simulink model "BLDCmotorControl_FOC_R2017b_fixdt"  (R2017b)
settings: Solver=FixedStepDiscrete  StartTime=0  StopTime=0.5  FixedStep=Ts  MaxStep=1e-6  RelTol=1e-6  AbsTol=1e-6  EnableMultiTasking=on
PreLoadFcn:
  | addpath(pwd);
  | addpath(genpath('01_Libraries'));
  | addpath(genpath('02_Figures'));
  | addpath(genpath('03_CreateParamTable'));
InitFcn:
  | init_model;
values from neighbouring files (symbols this model uses):
  a_elecAngle = 60    [init_model.m]
  a_elecPeriod = 360    [init_model.m]
  a_phaAdvMax = 25    [init_model.m]
  b_diagEna = 1    [init_model.m]
  b_fieldWeakEna = 0    [init_model.m]
  cf_currFilt = 0.12    [init_model.m]
  cf_idKi = 60 / (f_ctrl/3)    (= 0.01125)    [init_model.m]
  cf_idKp = 0.2    [init_model.m]
  cf_iqKi = 100 / (f_ctrl/3)    (= 0.01875)    [init_model.m]
  cf_iqKiLimProt = 60 / (f_ctrl/3)    (= 0.01125)    [init_model.m]
  cf_iqKp = 0.3    [init_model.m]
  cf_KbLimProt = 1000 / (f_ctrl/3)    (= 0.1875)    [init_model.m]
  cf_nKi = 20.4 / (f_ctrl/3)    (= 0.003825)    [init_model.m]
  cf_nKiLimProt = 20 / (f_ctrl/3)    (= 0.00375)    [init_model.m]
  cf_nKp = 1.18    [init_model.m]
  cf_speedCoef = round(f_ctrl * a_mechAngle * (pi/180) * (30/pi))    [init_model.m]
  CTRL_COM = 0    [init_model.m]
  CTRL_FOC = 2    [init_model.m]
  CTRL_SIN = 1    [init_model.m]
  dV_openRate = 1000 / (f_ctrl/3)    (= 0.1875)    [init_model.m]
  dz_cntTrnsDetHi = 40    [init_model.m]
  dz_cntTrnsDetLo = 20    [init_model.m]
  i_max = i_max * i_sca    (= 750)    [init_model.m]
  id_fieldWeakMax = 5 * i_sca    (= 250)    [init_model.m]
  iq_maxSca_M1 = sqrt(1 - iq_maxSca_XA.^2)    [init_model.m]
  n_commAcvLo = 15    [init_model.m]
  n_commDeacvHi = 30    [init_model.m]
  n_fieldWeakAuthHi = 400    [init_model.m]
  n_fieldWeakAuthLo = 300    [init_model.m]
  n_max = 1000    [init_model.m]
  n_polePairs = 15    [init_model.m]
  n_stdStillDet = 3    [init_model.m]
  OPEN_MODE = 0    [init_model.m]
  r_cos_M1 = cos((a_elecAngle_XA + 0)*(pi/180))    [init_model.m]
  r_errInpTgtThres = 600    [init_model.m]
  r_fieldWeakHi = 1500    [init_model.m]
  r_fieldWeakLo = 1000    [init_model.m]
  r_sin3PhaA_M1 = sin3Arm + A*r_sinPhaA_M1    [init_model.m]
  r_sin3PhaB_M1 = sin3Arm + A*r_sinPhaB_M1    [init_model.m]
  r_sin3PhaC_M1 = sin3Arm + A*r_sinPhaC_M1    [init_model.m]
  r_sin_M1 = sin((a_elecAngle_XA + 0)*(pi/180))    [init_model.m]
  SPD_MODE = 2    [init_model.m]
  t_errDequal = 1.80 * f_ctrl/3    (= 9600)    [init_model.m]
  t_errQual = 0.24 * f_ctrl/3    (= 1280)    [init_model.m]
  TRQ_MODE = 3    [init_model.m]
  Ts = 5e-6    (= 5e-06)    [init_model.m]
  Ts_ctrl = 6e-5    (= 6e-05)    [init_model.m]
  Vd_max = 1000 - V_margin    (= 900)    [init_model.m]
  vec_hallToPos = [0 2 0 1 4 3 5 0]    [init_model.m]
  VLT_MODE = 1    [init_model.m]
  Vq_max_M1 = sqrt(Vd_max^2 - Vq_max_XA.^2)    [init_model.m]
  z_commutMap_M1 = [-1 -1  0  1  1  0 ... (first row only)    [init_model.m]
  z_ctrlModReq = VLT_MODE    (= 1)    [init_model.m]
  z_ctrlTypSel = 2    [init_model.m]
  z_maxCntRst = 2000    [init_model.m]
  z_selPhaCurMeasABC = 0    [init_model.m]
undefined symbols (not defined in the file or in its folder): DiscIntNeverNeededParam, sigbuilder_block
libraries: BLDC_controller_Lib x15, simulink x14, powerlib x6, pePwmGenerator x1
(part 2 of 4)

== system BLDCmotorControl_FOC_R2017b_fixdt/rateLimiter ==
  u : Inport
  rate : Inport  Port=2
  Data Type Conversion1 : DataTypeConversion  OutDataTypeStr=fixdt(1,16,4)
  Gain : Gain  Tag=struct('comment',struct('text','','placement',1),'logdata',struct('maxnumvals',inf,'plotchannels',[],'loggingmode',3,'channels',1),'output',struct('variable','','description','','name','$S_$B','width',1,'address','','max',NaN,'min',NaN,'class','default','type','CONTINUOUS','scaling','','lsb',1,'offset',0,'arb',0,'freeze',1,'unit','','autoscalingmode',1,'lowerheadroom',1,'upperheadroom',1,'headroomunit','bit','keepdatatype',1,'checkmin',0,'checkmax',0,'castoutput',0,'show',0),'gain',struct('variable','','description','','name','$S_$B_gain','width',1,'address','','max',NaN,'min',NaN,'class','default','type','CONTINUOUS','scaling','','lsb',1,'offset',0,'arb',0,'freeze',1,'unit','','keepdatatype',1,'value','1','scalar',0,'tolerance',1),'scalingvalid',0,'date',730486)  Gain=-1  RndMeth=Zero  OutDataTypeStr=Inherit: Same as input  ParamDataTypeStr=Inherit: Same as input
  Rate_Limiter : Subsystem
      settings: RTWFcnNameOpts=Use subsystem name
      mask Display: plot([0.15 0.85],[0.5 0.5],[0.5 0.5],[0.1 0.9],[0.25 0.75],[0.1 0.9])
  y : Outport
  wires:
  Data Type Conversion1/1 -> Rate_Limiter/1(u)
  u/1 -> Data Type Conversion1/1
  Rate_Limiter/1(y) -> y/1
  rate/1 -> Gain/1, Rate_Limiter/2(inc)
  Gain/1 -> Rate_Limiter/3(dec)

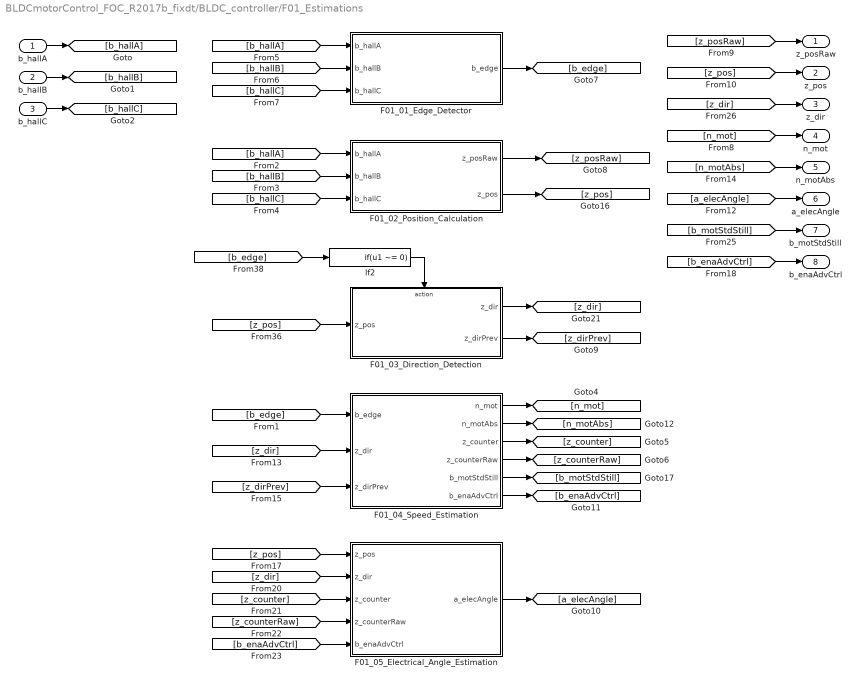
== system BLDCmotorControl_FOC_R2017b_fixdt/BLDC_controller/F01_Estimations ==
  b_hallA : Inport
  b_hallB : Inport  Port=2
  b_hallC : Inport  Port=3
  F01_01_Edge_Detector : Subsystem
  F01_02_Position_Calculation : Subsystem
  F01_03_Direction_Detection : Subsystem
  F01_04_Speed_Estimation : Subsystem
  F01_05_Electrical_Angle_Estimation : Subsystem
  If2 : If  IfExpression=u1 ~= 0  ShowElse=off
  z_posRaw : Outport  OutputWhenDisabled=reset  InitialOutput=0
  z_pos : Outport  Port=2  OutputWhenDisabled=reset  InitialOutput=0
  z_dir : Outport  Port=3  OutputWhenDisabled=reset  InitialOutput=0
  "n_mot " : Outport  Port=4  OutputWhenDisabled=reset  InitialOutput=0
  n_motAbs : Outport  Port=5  OutputWhenDisabled=reset  InitialOutput=0
  a_elecAngle : Outport  Port=6  OutputWhenDisabled=reset  InitialOutput=0
  b_motStdStill : Outport  Port=7  OutputWhenDisabled=reset  InitialOutput=0
  b_enaAdvCtrl : Outport  Port=8
  wires:
  If2/1 -> F01_03_Direction_Detection/Action
  [b_edge] -> If2/1
  [z_pos] -> F01_03_Direction_Detection/1(z_pos)
  [b_hallA] -> F01_01_Edge_Detector/1(b_hallA)
  F01_01_Edge_Detector/1("b_edge ") -> [b_edge]
  F01_03_Direction_Detection/1(z_dir) -> [z_dir]
  [b_hallB] -> F01_01_Edge_Detector/2(b_hallB)
  [b_hallC] -> F01_01_Edge_Detector/3(b_hallC)
  b_hallA/1 -> [b_hallA]
  b_hallB/1 -> [b_hallB]
  b_hallC/1 -> [b_hallC]
  [b_hallC] -> F01_02_Position_Calculation/3(b_hallC)
  [b_hallB] -> F01_02_Position_Calculation/2(b_hallB)
  [b_hallA] -> F01_02_Position_Calculation/1(b_hallA)
  F01_02_Position_Calculation/2("z_pos ") -> [z_pos]
  [b_edge] -> F01_04_Speed_Estimation/1(b_edge)
  F01_04_Speed_Estimation/1(n_mot) -> [n_mot]
  [n_mot] -> "n_mot "/1
  [z_pos] -> z_pos/1
  [z_dir] -> F01_04_Speed_Estimation/2(z_dir)
  F01_04_Speed_Estimation/3(z_counter) -> [z_counter]
  F01_04_Speed_Estimation/4(z_counterRaw) -> [z_counterRaw]
  F01_03_Direction_Detection/2(z_dirPrev) -> [z_dirPrev]
  [z_dirPrev] -> F01_04_Speed_Estimation/3(z_dirPrev)
  [z_pos] -> F01_05_Electrical_Angle_Estimation/1(z_pos)
  [z_dir] -> F01_05_Electrical_Angle_Estimation/2(z_dir)
  [z_counter] -> F01_05_Electrical_Angle_Estimation/3(z_counter)
  [z_counterRaw] -> F01_05_Electrical_Angle_Estimation/4(z_counterRaw)
  [b_enaAdvCtrl] -> F01_05_Electrical_Angle_Estimation/5(b_enaAdvCtrl)
  F01_04_Speed_Estimation/6(b_enaAdvCtrl) -> [b_enaAdvCtrl]
  [b_enaAdvCtrl] -> b_enaAdvCtrl/1
  [a_elecAngle] -> a_elecAngle/1
  F01_05_Electrical_Angle_Estimation/1(a_elecAngle) -> [a_elecAngle]
  F01_04_Speed_Estimation/2(n_motAbs) -> [n_motAbs]
  [n_motAbs] -> n_motAbs/1
  F01_02_Position_Calculation/1(z_posRaw) -> [z_posRaw]
  [z_posRaw] -> z_posRaw/1
  [b_motStdStill] -> b_motStdStill/1
  F01_04_Speed_Estimation/5(b_motStdStill) -> [b_motStdStill]
  [z_dir] -> z_dir/1

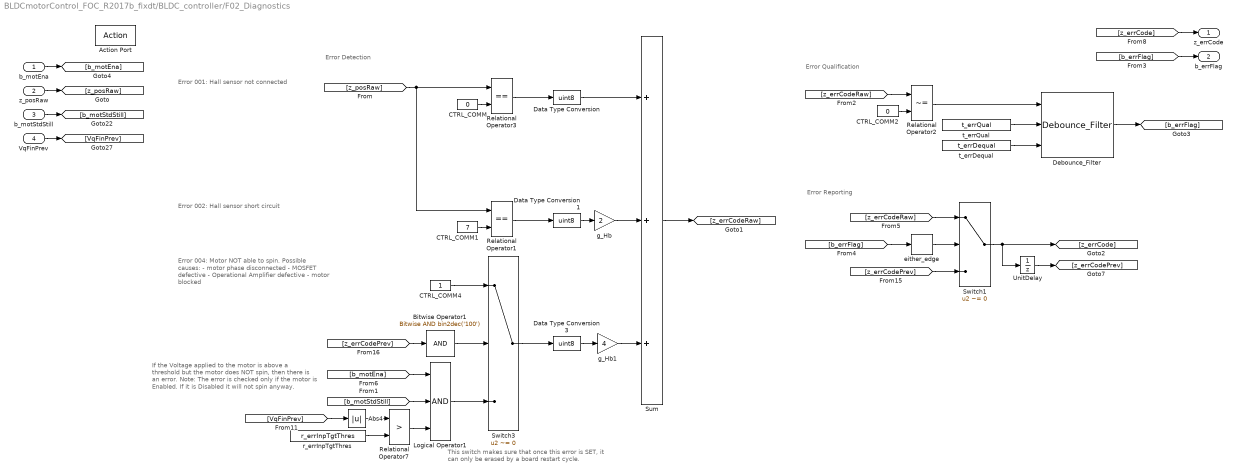
== system BLDCmotorControl_FOC_R2017b_fixdt/BLDC_controller/F02_Diagnostics ==
  note: Error 001: Hall sensor not connected
  note: Error 002: Hall sensor short circuit
  note: Error Qualification
  note: Error Detection
  note: Error Reporting
  note: Error 004: Motor NOT able to spin.
      |
      | Possible causes:
      | - motor phase disconnected
      | - MOSFET defective
      | - Operational Amplifier defective
      | - motor blocked
  note: This switch makes sure that once this error is SET, it can only be erased by a board restart cycle.
  note: If the Voltage applied to the motor is above a threshold but the motor does NOT spin, then there is an error.
      | Note: The error is checked only if the motor is Enabled. If it is Disabled it will not spin anyway.
  b_motEna : Inport
  z_posRaw : Inport  Port=2
  b_motStdStill : Inport  Port=3
  VqFinPrev : Inport  Port=4
  Action Port : ActionPort  ActionType=then
  Abs4 : Abs
  Bitwise Operator1 : simulink/Logic and Bit Operations/Bitwise Operator  logicop=AND  UseBitMask=on  BitMask=bin2dec('100')  BitMaskRealWorld=Stored Integer
  CTRL_COMM : Constant  Value=0  OutDataTypeStr=Inherit: Inherit via back propagation
  CTRL_COMM1 : Constant  Value=7  OutDataTypeStr=Inherit: Inherit via back propagation
  CTRL_COMM2 : Constant  Value=0  OutDataTypeStr=Inherit: Inherit via back propagation
  CTRL_COMM4 : Constant  OutDataTypeStr=Inherit: Inherit via back propagation
  Data Type Conversion : DataTypeConversion  OutDataTypeStr=uint8
  Data Type Conversion1 : DataTypeConversion  OutDataTypeStr=uint8
  Data Type Conversion3 : DataTypeConversion  OutDataTypeStr=uint8
  Debounce_Filter : BLDC_controller_Lib/Debounce_Filter
  Logical Operator1 : Logic  Inputs=3  AllPortsSameDT=off  OutDataTypeStr=boolean
  Relational Operator1 : RelationalOperator  Operator===  OutDataTypeStr=boolean  RndMeth=Simplest
  Relational Operator2 : RelationalOperator  Operator=~=  OutDataTypeStr=boolean  RndMeth=Simplest
  Relational Operator3 : RelationalOperator  Operator===  OutDataTypeStr=boolean  RndMeth=Simplest
  Relational Operator7 : RelationalOperator  Operator=>  OutDataTypeStr=boolean  RndMeth=Simplest
  Sum : Sum  Inputs=+++  RndMeth=Simplest  OutDataTypeStr=Inherit: Same as first input
  Switch1 : Switch  Criteria=u2 ~= 0  OutDataTypeStr=Inherit: Inherit via back propagation  RndMeth=Zero
  Switch3 : Switch  Criteria=u2 ~= 0  OutDataTypeStr=Inherit: Inherit via back propagation  RndMeth=Zero
  UnitDelay : UnitDelay  SampleTime=-1
      settings: AttributesFormatString=Ini=%<X0>
  either_edge : BLDC_controller_Lib/either_edge
  g_Hb : Gain  Gain=2  RndMeth=Simplest  OutDataTypeStr=Inherit: Same as input
  g_Hb1 : Gain  Gain=4  RndMeth=Simplest  OutDataTypeStr=Inherit: Same as input
  r_errInpTgtThres : Constant  Value=r_errInpTgtThres  OutDataTypeStr=Inherit: Inherit via back propagation
  t_errDequal : Constant  Value=t_errDequal  OutDataTypeStr=Inherit: Inherit via back propagation
  t_errQual : Constant  Value=t_errQual  OutDataTypeStr=Inherit: Inherit via back propagation
  "z_errCode " : Outport
  b_errFlag : Outport  Port=2
  wires:
  [z_errCode] -> "z_errCode "/1
  z_posRaw/1 -> [z_posRaw]
  t_errDequal/1 -> Debounce_Filter/3
  t_errQual/1 -> Debounce_Filter/2
  CTRL_COMM/1 -> Relational Operator3/2
  CTRL_COMM1/1 -> Relational Operator1/2
  [z_posRaw] -> Relational Operator1/1, Relational Operator3/1
  Relational Operator3/1 -> Data Type Conversion/1
  Sum/1 -> [z_errCodeRaw]
  Relational Operator2/1 -> Debounce_Filter/1
  [z_errCodeRaw] -> Relational Operator2/1
  CTRL_COMM2/1 -> Relational Operator2/2
  Debounce_Filter/1 -> [b_errFlag]
  either_edge/1 -> Switch1/2
  Switch1/1 -> [z_errCode], UnitDelay/1
  [b_errFlag] -> b_errFlag/1
  [b_errFlag] -> either_edge/1
  [z_errCodeRaw] -> Switch1/1
  g_Hb/1 -> Sum/2
  Relational Operator1/1 -> Data Type Conversion1/1
  Data Type Conversion/1 -> Sum/1
  Data Type Conversion1/1 -> g_Hb/1
  Switch3/1 -> Data Type Conversion3/1
  Data Type Conversion3/1 -> g_Hb1/1
  g_Hb1/1 -> Sum/3
  VqFinPrev/1 -> [VqFinPrev]
  b_motStdStill/1 -> [b_motStdStill]
  [VqFinPrev] -> Abs4/1
  Abs4/1 -> Relational Operator7/1
  r_errInpTgtThres/1 -> Relational Operator7/2
  UnitDelay/1 -> [z_errCodePrev]
  [z_errCodePrev] -> Switch1/3
  [z_errCodePrev] -> Bitwise Operator1/1
  Bitwise Operator1/1 -> Switch3/2
  CTRL_COMM4/1 -> Switch3/1
  Logical Operator1/1 -> Switch3/3
  b_motEna/1 -> [b_motEna]
  Relational Operator7/1 -> Logical Operator1/3
  [b_motEna] -> Logical Operator1/1
  [b_motStdStill] -> Logical Operator1/2

== system BLDCmotorControl_FOC_R2017b_fixdt/BLDC_controller/F03_Control_Mode_Manager ==
  b_errFlag : Inport
  b_motEna : Inport  Port=2
  z_ctrlTypSel : Inport  Port=3
  z_ctrlModReq : Inport  Port=4
  r_inpTgt : Inport  Port=5
  VqFinPrev : Inport  Port=6
  Action Port : ActionPort  ActionType=then
  F03_01_Mode_Transition_Calculation : Subsystem
  F03_02_Control_Mode_Manager : Stateflow chart  TreatAsAtomicUnit=on
  F03_03_Input_Target_Synthesis : Subsystem
  z_ctrlMod : Outport
  r_inpTgtSca : Outport  Port=2
  wires:
  [z_ctrlMod] -> z_ctrlMod/1
  b_motEna/1 -> [b_motEna]
  [b_toOpen] -> F03_02_Control_Mode_Manager/1(b_toOpen)
  [b_toSpdMod] -> F03_02_Control_Mode_Manager/3(b_toSpdMod)
  z_ctrlModReq/1 -> [z_ctrlModReq]
  [b_toTrqMod] -> F03_02_Control_Mode_Manager/4(b_toTrqMod)
  F03_02_Control_Mode_Manager/1(z_ctrlMod) -> [z_ctrlMod]
  [b_toActive] -> F03_02_Control_Mode_Manager/2(b_toActive)
  F03_01_Mode_Transition_Calculation/1(b_toOpen) -> [b_toOpen]
  F03_01_Mode_Transition_Calculation/2(b_toActive) -> [b_toActive]
  F03_01_Mode_Transition_Calculation/3(b_toSpdMod) -> [b_toSpdMod]
  F03_01_Mode_Transition_Calculation/4(b_toTrqMod) -> [b_toTrqMod]
  [b_motEna] -> F03_01_Mode_Transition_Calculation/1(b_motEna)
  [z_ctrlModReq] -> F03_01_Mode_Transition_Calculation/3(z_ctrlModReq)
  b_errFlag/1 -> [b_errFlag]
  [b_errFlag] -> F03_01_Mode_Transition_Calculation/2(b_errFlag)
  [z_ctrlModReq] -> F03_03_Input_Target_Synthesis/2(z_ctrlModReq)
  [z_ctrlTypSel] -> F03_03_Input_Target_Synthesis/1(z_ctrlTypSel)
  [r_inpTgt] -> F03_03_Input_Target_Synthesis/4(r_inpTgt)
  F03_03_Input_Target_Synthesis/1(r_inpTgtSca) -> [r_inpTgtSca]
  [z_ctrlMod] -> F03_03_Input_Target_Synthesis/3(z_ctrlMod)
  VqFinPrev/1 -> [VqFinPrev]
  [VqFinPrev] -> F03_03_Input_Target_Synthesis/5(VqFinPrev)
  r_inpTgt/1 -> [r_inpTgt]
  z_ctrlTypSel/1 -> [z_ctrlTypSel]
  [r_inpTgtSca] -> r_inpTgtSca/1

== system BLDCmotorControl_FOC_R2017b_fixdt/BLDC_controller/F04_Field_Weakening ==
  note: Calculate Blending Factor
  note: This blendig factor is a number between [0, 1]. It manages the Field weakening amount, ranging from 0 to a calibratable Max value.
  note: Field Weakening / Phase Advance
  z_ctrlTypSel : Inport
  r_inpTgt : Inport  Port=2
  n_motAbs : Inport  Port=3
  Action Port : ActionPort  ActionType=then
  Abs5 : Abs  OutDataTypeStr=Inherit: Inherit via back propagation  RndMeth=Zero
  CTRL_COMM2 : Constant  Value=CTRL_FOC  OutDataTypeStr=Inherit: Inherit via back propagation
  Divide1 : Product  Inputs=*/  OutDataTypeStr=fixdt(0,16,15)  RndMeth=Simplest
  Divide14 : Product  Inputs=*/  OutDataTypeStr=fixdt(0,16,15)  RndMeth=Simplest
  Divide2 : Product  Inputs=**  OutDataTypeStr=fixdt(0,16,15)  RndMeth=Simplest
  Divide3 : Product  Inputs=**  RndMeth=Simplest  OutDataTypeStr=Inherit: Same as first input
  Relational Operator1 : RelationalOperator  Operator===  OutDataTypeStr=boolean  RndMeth=Simplest
  Saturation Dynamic : simulink/Discontinuities/Saturation Dynamic  OutMin=[]  OutMax=[]  OutDataTypeStr=Inherit: Same as second input  OutDataType=fixdt(1, 16)  OutScaling=2^-10  DoSatur=off
  Saturation Dynamic1 : simulink/Discontinuities/Saturation Dynamic  OutMin=[]  OutMax=[]  OutDataTypeStr=Inherit: Same as second input  OutDataType=fixdt(1, 16)  OutScaling=2^-10  DoSatur=off
  Sum{1..4} (4 alike) : Sum  Inputs=+-  RndMeth=Simplest  OutDataTypeStr=Inherit: Same as first input
  Switch2 : Switch  Criteria=u2 ~= 0  OutDataTypeStr=Inherit: Inherit via back propagation  RndMeth=Zero
  a_phaAdvMax : Constant  Value=a_phaAdvMax  OutDataTypeStr=fixdt(1,16,4)
  id_fieldWeakMax : Constant  Value=id_fieldWeakMax  OutDataTypeStr=fixdt(1,16,4)
  n_fieldWeakAuthHi : Constant  Value=n_fieldWeakAuthHi  OutDataTypeStr=fixdt(1,16,4)
  n_fieldWeakAuthLo : Constant  Value=n_fieldWeakAuthLo  OutDataTypeStr=fixdt(1,16,4)
  r_fieldWeakHi : Constant  Value=r_fieldWeakHi  OutDataTypeStr=fixdt(1,16,4)
  r_fieldWeakLo : Constant  Value=r_fieldWeakLo  OutDataTypeStr=fixdt(1,16,4)
  "r_fieldWeak " : Outport
  wires:
  a_phaAdvMax/1 -> Switch2/3
  [r_fieldWeak] -> "r_fieldWeak "/1
  Switch2/1 -> Divide3/1
  n_fieldWeakAuthLo/1 -> Saturation Dynamic/3, Sum4/2, Sum2/2
  CTRL_COMM2/1 -> Relational Operator1/2
  Relational Operator1/1 -> Switch2/2
  [n_motAbs] -> Saturation Dynamic/2
  n_motAbs/1 -> [n_motAbs]
  Divide14/1 -> Divide2/1
  Saturation Dynamic/1 -> Sum4/1
  n_fieldWeakAuthHi/1 -> Saturation Dynamic/1, Sum2/1
  Divide1/1 -> Divide2/2
  Sum4/1 -> Divide1/1
  [r_blendFactor] -> Divide3/2
  Sum3/1 -> Divide14/2
  id_fieldWeakMax/1 -> Switch2/1
  [r_inpTgt] -> Abs5/1
  Saturation Dynamic1/1 -> Sum1/1
  Divide2/1 -> [r_blendFactor]
  Sum2/1 -> Divide1/2
  Abs5/1 -> Saturation Dynamic1/2
  z_ctrlTypSel/1 -> [z_ctrlTypSel]
  r_inpTgt/1 -> [r_inpTgt]
  r_fieldWeakHi/1 -> Saturation Dynamic1/1, Sum3/1
  r_fieldWeakLo/1 -> Saturation Dynamic1/3, Sum3/2, Sum1/2
  Divide3/1 -> [r_fieldWeak]
  Sum1/1 -> Divide14/1
  [z_ctrlTypSel] -> Relational Operator1/1

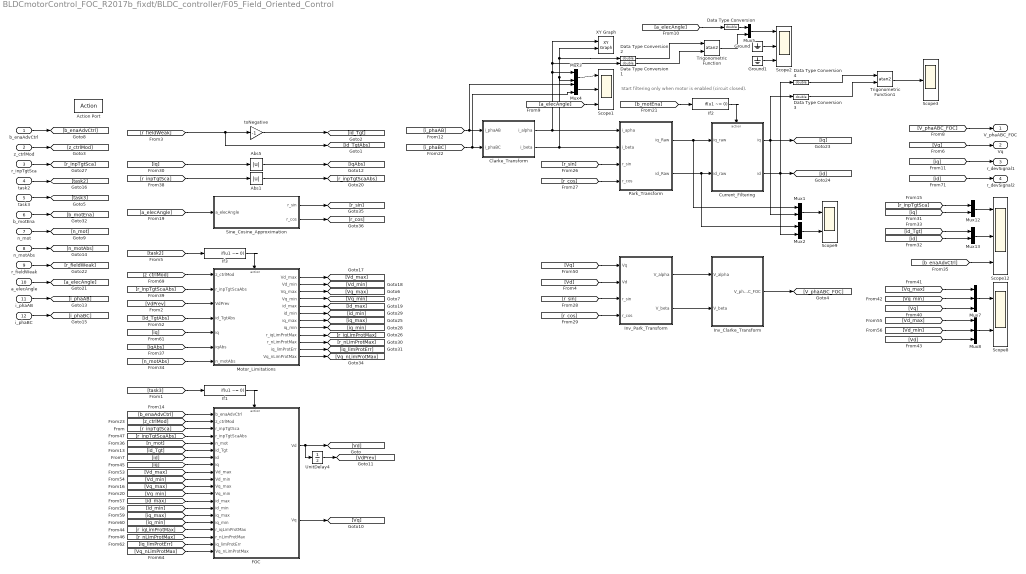
== system BLDCmotorControl_FOC_R2017b_fixdt/BLDC_controller/F05_Field_Oriented_Control ==
  note: Start filtering only when motor is enabled (circuit closed).
  b_enaAdvCtrl : Inport
  z_ctrlMod : Inport  Port=2
  r_inpTgtSca : Inport  Port=3
  task2 : Inport  Port=4
  task3 : Inport  Port=5
  b_motEna : Inport  Port=6
  n_mot : Inport  Port=7
  n_motAbs : Inport  Port=8
  r_fieldWeak : Inport  Port=9
  a_elecAngle : Inport  Port=10
  i_phaAB : Inport  Port=11
  i_phaBC : Inport  Port=12
  Action Port : ActionPort  InitializeStates=reset  ActionType=then
  Abs1 : Abs  OutDataTypeStr=Inherit: Inherit via back propagation  RndMeth=Zero
  Abs5 : Abs  OutDataTypeStr=Inherit: Inherit via back propagation  RndMeth=Zero
  Clarke_Transform : Subsystem
  Current_Filtering : Subsystem
  Data Type Conversion{,1..4} (5 alike) : DataTypeConversion  OutDataTypeStr=double
  FOC : Subsystem
  Ground : Ground
  Ground1 : Ground
  If1 : If  IfExpression=u1 ~= 0  ShowElse=off
  If2 : If  IfExpression=u1 ~= 0  ShowElse=off
  If3 : If  IfExpression=u1 ~= 0  ShowElse=off
  Inv_Clarke_Transform : Subsystem
  Inv_Park_Transform : Subsystem
  Motor_Limitations : Subsystem
  Mux{1..5,12..13} (7 alike) : Mux  Inputs=2
  Mux7 : Mux  Inputs=3
  Mux8 : Mux  Inputs=3
  Park_Transform : Subsystem
  Scope1 : Scope  NumInputPorts=3
  Scope12 : Scope  NumInputPorts=3
  Scope2 : Scope  NumInputPorts=3
  Scope3 : Scope
  Scope8 : Scope  NumInputPorts=2
  Scope9 : Scope  NumInputPorts=2
  Sine_Cosine_Approximation : Subsystem
  Trigonometric Function : Trigonometry  Operator=atan2  NumberOfIterations=5
  Trigonometric Function1 : Trigonometry  Operator=atan2  NumberOfIterations=5
  UnitDelay4 : UnitDelay  SampleTime=-1
      settings: AttributesFormatString=Ini=%<X0>
  XY Graph : simulink/Sinks/XY Graph  xmin=-1000  xmax=1000  ymin=-1000  ymax=1000  st=-1
  toNegative : Gain  Tag=struct('comment',struct('text','','placement',1),'logdata',struct('maxnumvals',inf,'plotchannels',[],'loggingmode',3,'channels',1),'output',struct('variable','','description','','name','$S_$B','width',1,'address','','max',NaN,'min',NaN,'class','default','type','CONTINUOUS','scaling','','lsb',1,'offset',0,'arb',0,'freeze',1,'unit','','autoscalingmode',1,'lowerheadroom',1,'upperheadroom',1,'headroomunit','bit','keepdatatype',1,'checkmin',0,'checkmax',0,'castoutput',0,'show',0),'gain',struct('variable','','description','','name','$S_$B_gain','width',1,'address','','max',NaN,'min',NaN,'class','default','type','CONTINUOUS','scaling','','lsb',1,'offset',0,'arb',0,'freeze',1,'unit','','keepdatatype',1,'value','1','scalar',0,'tolerance',1),'scalingvalid',0,'date',730486)  Gain=-1  RndMeth=Zero  OutDataTypeStr=Inherit: Same as input  ParamDataTypeStr=Inherit: Same as input
  V_phaABC_FOC : Outport  OutputWhenDisabled=reset  InitialOutput=0
  Vq : Outport  Port=2  InitialOutput=0
  r_devSignal1 : Outport  Port=3  OutputWhenDisabled=reset  InitialOutput=0
  r_devSignal2 : Outport  Port=4  OutputWhenDisabled=reset  InitialOutput=0
  wires:
  [V_phaABC_FOC] -> V_phaABC_FOC/1
  Inv_Park_Transform/1(V_alpha) -> Inv_Clarke_Transform/1(V_alpha)
  Inv_Park_Transform/2(V_beta) -> Inv_Clarke_Transform/2(V_beta)
  i_phaAB/1 -> [i_phaAB]
  i_phaBC/1 -> [i_phaBC]
  Inv_Clarke_Transform/1(V_phaABC_FOC) -> [V_phaABC_FOC]
  Clarke_Transform/2(i_beta) -> Data Type Conversion2/1, XY Graph/2, Mux3/2, Park_Transform/2(i_beta)
  Mux12/1 -> Scope12/1
  Mux13/1 -> Scope12/2
  [r_sin] -> Park_Transform/3(r_sin)
  [r_cos] -> Park_Transform/4(r_cos)
  [r_sin] -> Inv_Park_Transform/3(r_sin)
  [r_cos] -> Inv_Park_Transform/4(r_cos)
  [r_inpTgtSca] -> Mux12/1
  [iq] -> Mux12/2
  [id] -> Mux13/2
  [id_Tgt] -> Mux13/1
  r_inpTgtSca/1 -> [r_inpTgtSca]
  [i_phaAB] -> Mux4/1, Clarke_Transform/1(i_phaAB)
  [i_phaBC] -> Mux4/2, Clarke_Transform/2(i_phaBC)
  [Vd_max] -> Mux8/1
  [Vd] -> Mux8/3
  Mux8/1 -> Scope8/2
  [Vd_min] -> Mux8/2
  [Vq] -> Mux7/3
  Mux7/1 -> Scope8/1
  [Vq_max] -> Mux7/1
  [Vq_min] -> Mux7/2
  Park_Transform/2(id_Raw) -> Current_Filtering/2(id_raw), Mux2/1
  Park_Transform/1(iq_Raw) -> Current_Filtering/1(iq_raw), Mux1/1
  Current_Filtering/1(iq) -> Data Type Conversion3/1, [iq], Mux1/2
  Current_Filtering/2(id) -> Data Type Conversion4/1, [id], Mux2/2
  [Vq] -> Vq/1
  b_enaAdvCtrl/1 -> [b_enaAdvCtrl]
  [Vd] -> Inv_Park_Transform/2(Vd)
  z_ctrlMod/1 -> [z_ctrlMod]
  n_mot/1 -> [n_mot]
  [b_enaAdvCtrl] -> Scope12/3
  [Vq] -> Inv_Park_Transform/1(Vq)
  Motor_Limitations/3(Vq_max) -> [Vq_max]
  Motor_Limitations/4(Vq_min) -> [Vq_min]
  [VdPrev] -> Motor_Limitations/3(VdPrev)
  [id_TgtAbs] -> Motor_Limitations/4(id_TgtAbs)
  Motor_Limitations/2(Vd_min) -> [Vd_min]
  Motor_Limitations/1(Vd_max) -> [Vd_max]
  Motor_Limitations/5(id_max) -> [id_max]
  Motor_Limitations/6(id_min) -> [id_min]
  Motor_Limitations/7(iq_max) -> [iq_max]
  Motor_Limitations/8(iq_min) -> [iq_min]
  [iq] -> Motor_Limitations/5(iq)
  Motor_Limitations/11(iq_limProtErr) -> [iq_limProtErr]
  Motor_Limitations/12(Vq_nLimProtMax) -> [Vq_nLimProtMax]
  [z_ctrlMod] -> Motor_Limitations/1(z_ctrlMod)
  r_fieldWeak/1 -> [r_fieldWeak]
  Sine_Cosine_Approximation/1(r_sin) -> [r_sin]
  Sine_Cosine_Approximation/2(r_cos) -> [r_cos]
  [a_elecAngle] -> Sine_Cosine_Approximation/1(a_elecAngle)
  a_elecAngle/1 -> [a_elecAngle]
  Mux1/1 -> Scope9/1
  Mux2/1 -> Scope9/2
  [id] -> r_devSignal2/1
  [iq] -> r_devSignal1/1
  If2/1 -> Current_Filtering/Action
  b_motEna/1 -> [b_motEna]
  [b_motEna] -> If2/1
  toNegative/1 -> [id_Tgt]
  [r_fieldWeak] -> toNegative/1, [id_TgtAbs]
  task2/1 -> [task2]
  task3/1 -> [task3]
  If3/1 -> Motor_Limitations/Action
  [task2] -> If3/1
  If1/1 -> FOC/Action
  [task3] -> If1/1
  FOC/2(Vq) -> [Vq]
  [b_enaAdvCtrl] -> FOC/1(b_enaAdvCtrl)
  [id_Tgt] -> FOC/6(id_Tgt)
  [id] -> FOC/7(id)
  [Vd_max] -> FOC/9(Vd_max)
  [Vd_min] -> FOC/10(Vd_min)
  [id_max] -> FOC/13(id_max)
  [id_min] -> FOC/14(id_min)
  [r_inpTgtSca] -> FOC/3(r_inpTgtSca)
  [Vq_max] -> FOC/11(Vq_max)
  [Vq_min] -> FOC/12(Vq_min)
  [iq_limProtErr] -> FOC/19(iq_limProtErr)
  [Vq_nLimProtMax] -> FOC/20(Vq_nLimProtMax)
  [iq_max] -> FOC/15(iq_max)
  [iq_min] -> FOC/16(iq_min)
  [iq] -> FOC/8(iq)
  [n_mot] -> FOC/5(n_mot)
  [z_ctrlMod] -> FOC/2(z_ctrlMod)
  FOC/1(Vd) -> UnitDelay4/1, [Vd]
  UnitDelay4/1 -> [VdPrev]
  Abs5/1 -> [iqAbs]
  [iq] -> Abs5/1
  n_motAbs/1 -> [n_motAbs]
  [n_motAbs] -> Motor_Limitations/7(n_motAbs)
  [iqAbs] -> Motor_Limitations/6(iqAbs)
  [r_inpTgtSca] -> Abs1/1
  Abs1/1 -> [r_inpTgtScaAbs]
  [r_inpTgtScaAbs] -> Motor_Limitations/2(r_inpTgtScaAbs)
  Motor_Limitations/9(r_iqLimProtMax) -> [r_iqLimProtMax]
  [r_iqLimProtMax] -> FOC/17(r_iqLimProtMax)
  Motor_Limitations/10(r_nLimProtMax) -> [r_nLimProtMax]
  [r_nLimProtMax] -> FOC/18(r_nLimProtMax)
  [r_inpTgtScaAbs] -> FOC/4(r_inpTgtScaAbs)
  Mux3/1 -> Scope1/1
  Clarke_Transform/1(i_alpha) -> Data Type Conversion1/1, XY Graph/1, Mux3/1, Park_Transform/1(i_apha)
  [a_elecAngle] -> Scope1/3
  Mux4/1 -> Scope1/2
  Mux5/1 -> Scope2/1
  Data Type Conversion/1 -> Mux5/1
  [a_elecAngle] -> Data Type Conversion/1
  Trigonometric Function/1 -> Mux5/2
  Ground/1 -> Scope2/2
  Ground1/1 -> Scope2/3
  Data Type Conversion2/1 -> Trigonometric Function/1
  Data Type Conversion1/1 -> Trigonometric Function/2
  Data Type Conversion3/1 -> Trigonometric Function1/2
  Data Type Conversion4/1 -> Trigonometric Function1/1
  Trigonometric Function1/1 -> Scope3/1

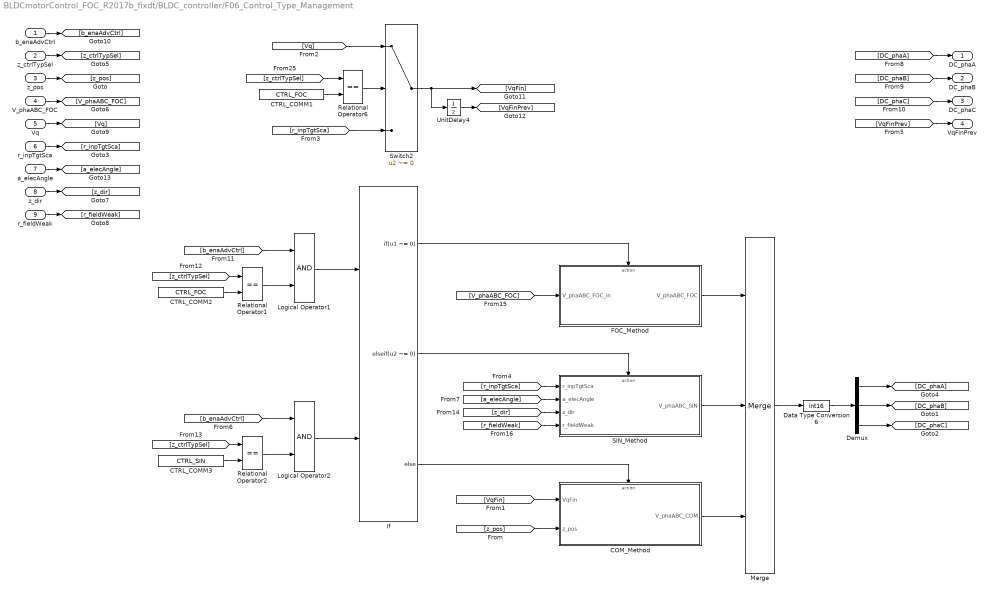
== system BLDCmotorControl_FOC_R2017b_fixdt/BLDC_controller/F06_Control_Type_Management ==
  b_enaAdvCtrl : Inport
  z_ctrlTypSel : Inport  Port=2
  z_pos : Inport  Port=3
  V_phaABC_FOC : Inport  Port=4
  Vq : Inport  Port=5
  r_inpTgtSca : Inport  Port=6
  a_elecAngle : Inport  Port=7
  z_dir : Inport  Port=8
  r_fieldWeak : Inport  Port=9
  COM_Method : Subsystem
  CTRL_COMM1 : Constant  Value=CTRL_FOC  OutDataTypeStr=Inherit: Inherit via back propagation
  CTRL_COMM2 : Constant  Value=CTRL_FOC  OutDataTypeStr=Inherit: Inherit via back propagation
  CTRL_COMM3 : Constant  Value=CTRL_SIN  OutDataTypeStr=Inherit: Inherit via back propagation
  Data Type Conversion6 : DataTypeConversion  OutDataTypeStr=int16
  Demux : Demux  Outputs=3
  FOC_Method : Subsystem
  If : If  NumInputs=2  IfExpression=u1 ~= 0  ElseIfExpressions=u2 ~= 0
  Logical Operator1 : Logic  AllPortsSameDT=off  OutDataTypeStr=boolean
  Logical Operator2 : Logic  AllPortsSameDT=off  OutDataTypeStr=boolean
  Merge : Merge  Inputs=3
  Relational Operator1 : RelationalOperator  Operator===  OutDataTypeStr=boolean  RndMeth=Simplest
  Relational Operator2 : RelationalOperator  Operator===  OutDataTypeStr=boolean  RndMeth=Simplest
  Relational Operator6 : RelationalOperator  Operator===  OutDataTypeStr=boolean  RndMeth=Simplest
  SIN_Method : Subsystem
  Switch2 : Switch  Criteria=u2 ~= 0  OutDataTypeStr=Inherit: Inherit via back propagation  RndMeth=Zero
  UnitDelay4 : UnitDelay  SampleTime=-1
      settings: AttributesFormatString=Ini=%<X0>
  DC_phaA : Outport  OutputWhenDisabled=reset  InitialOutput=0
  DC_phaB : Outport  Port=2  OutputWhenDisabled=reset  InitialOutput=0
  "DC_phaC " : Outport  Port=3  OutputWhenDisabled=reset  InitialOutput=0
  VqFinPrev : Outport  Port=4  OutputWhenDisabled=reset  InitialOutput=0
  wires:
  Demux/3 -> [DC_phaC]
  Demux/2 -> [DC_phaB]
  Demux/1 -> [DC_phaA]
  z_pos/1 -> [z_pos]
  [DC_phaC] -> "DC_phaC "/1
  [DC_phaB] -> DC_phaB/1
  [DC_phaA] -> DC_phaA/1
  Merge/1 -> Data Type Conversion6/1
  V_phaABC_FOC/1 -> [V_phaABC_FOC]
  Vq/1 -> [Vq]
  b_enaAdvCtrl/1 -> [b_enaAdvCtrl]
  [z_ctrlTypSel] -> Relational Operator6/1
  CTRL_COMM1/1 -> Relational Operator6/2
  Relational Operator6/1 -> Switch2/2
  r_inpTgtSca/1 -> [r_inpTgtSca]
  z_ctrlTypSel/1 -> [z_ctrlTypSel]
  Switch2/1 -> UnitDelay4/1, [VqFin]
  UnitDelay4/1 -> [VqFinPrev]
  [VqFinPrev] -> VqFinPrev/1
  [Vq] -> Switch2/1
  [r_inpTgtSca] -> Switch2/3
  Data Type Conversion6/1 -> Demux/1
  CTRL_COMM2/1 -> Relational Operator1/2
  [z_ctrlTypSel] -> Relational Operator1/1
  Relational Operator1/1 -> Logical Operator1/2
  [b_enaAdvCtrl] -> Logical Operator1/1
  [z_ctrlTypSel] -> Relational Operator2/1
  CTRL_COMM3/1 -> Relational Operator2/2
  [V_phaABC_FOC] -> FOC_Method/1(V_phaABC_FOC_in)
  If/3 -> COM_Method/Action
  COM_Method/1(V_phaABC_COM) -> Merge/3
  [z_pos] -> COM_Method/2(z_pos)
  [VqFin] -> COM_Method/1(VqFin)
  [r_inpTgtSca] -> SIN_Method/1(r_inpTgtSca)
  Logical Operator1/1 -> If/1
  If/2 -> SIN_Method/Action
  SIN_Method/1(V_phaABC_SIN) -> Merge/2
  FOC_Method/1(V_phaABC_FOC) -> Merge/1
  If/1 -> FOC_Method/Action
  Relational Operator2/1 -> Logical Operator2/2
  Logical Operator2/1 -> If/2
  [b_enaAdvCtrl] -> Logical Operator2/1
  a_elecAngle/1 -> [a_elecAngle]
  z_dir/1 -> [z_dir]
  r_fieldWeak/1 -> [r_fieldWeak]
  [a_elecAngle] -> SIN_Method/2(a_elecAngle)
  [z_dir] -> SIN_Method/3(z_dir)
  [r_fieldWeak] -> SIN_Method/4(r_fieldWeak)

== system BLDCmotorControl_FOC_R2017b_fixdt/BLDC_controller/Implemented_control_methods ==

== system BLDCmotorControl_FOC_R2017b_fixdt/BLDC_controller/Task_Scheduler ==
  note: Task Squeduler : This creates a pulse train for alternating task squeduling in series.
  Data Type Conversion : DataTypeConversion  OutDataTypeStr=boolean
  Logical Operator2 : Logic  Commented=on  Operator=NOT  AllPortsSameDT=off  OutDataTypeStr=boolean
  UnitDelay2 : UnitDelay  InitialCondition=1  SampleTime=-1
      settings: AttributesFormatString=Ini=%<X0>
  UnitDelay4 : UnitDelay  Commented=on  InitialCondition=1  SampleTime=-1
      settings: AttributesFormatString=Ini=%<X0>
  UnitDelay5 : UnitDelay  SampleTime=-1
      settings: AttributesFormatString=Ini=%<X0>
  UnitDelay6 : UnitDelay  SampleTime=-1
      settings: AttributesFormatString=Ini=%<X0>
  task1 : Outport  OutputWhenDisabled=reset  InitialOutput=0
  task2 : Outport  Port=2  OutputWhenDisabled=reset  InitialOutput=0
  task3 : Outport  Port=3  OutputWhenDisabled=reset  InitialOutput=0
  wires:
  Logical Operator2/1 -> UnitDelay4/1
  UnitDelay4/1 -> Logical Operator2/1
  UnitDelay2/1 -> task1/1, UnitDelay5/1
  UnitDelay6/1 -> task3/1, Data Type Conversion/1
  UnitDelay5/1 -> task2/1, UnitDelay6/1
  Data Type Conversion/1 -> UnitDelay2/1

== system BLDCmotorControl_FOC_R2017b_fixdt/BLDC_model_closed/__InputSSForSFun__ ==
  gates_PWM : Inport
  Tm_Nm : Inport  Port=2
  __UniqueOutportName__1__ : Outport
  __UniqueOutportName__2__ : Outport  Port=2
  wires:
  gates_PWM/1 -> __UniqueOutportName__1__/1
  Tm_Nm/1 -> __UniqueOutportName__2__/1

== system BLDCmotorControl_FOC_R2017b_fixdt/BLDC_model_closed/__OutputSSForSFun__ ==
  __UniqueInportName__1__ : Inport
  __UniqueInportName__2__ : Inport  Port=2
  __UniqueInportName__3__ : Inport  Port=3
  __UniqueInportName__4__ : Inport  Port=4
  __UniqueInportName__5__ : Inport  Port=5
  __UniqueInportName__6__ : Inport  Port=6
  __UniqueInportName__7__ : Inport  Port=7
  __UniqueInportName__8__ : Inport  Port=8
  __UniqueInportName__9__ : Inport  Port=9
  __UniqueInportName__10__ : Inport  Port=10
  __UniqueInportName__11__ : Inport  Port=11
  __UniqueInportName__12__ : Inport  Port=12
  Mux1 : BusCreator  Inputs=12
  motor_out : Outport
  wires:
  __UniqueInportName__1__/1 -> Mux1/1  "Stator current is_a (A)"
  __UniqueInportName__2__/1 -> Mux1/2  "Stator current is_b (A)"
  __UniqueInportName__3__/1 -> Mux1/3  "Stator current is_c (A)"
  __UniqueInportName__4__/1 -> Mux1/4  "Stator back EMF e_a (V)"
  __UniqueInportName__5__/1 -> Mux1/5  "Stator back EMF e_b (V)"
  __UniqueInportName__6__/1 -> Mux1/6  "Stator back EMF e_cV)"
  __UniqueInportName__7__/1 -> Mux1/7  "Hall effect signal h_a"
  __UniqueInportName__8__/1 -> Mux1/8  "Hall effect signal h_b"
  __UniqueInportName__9__/1 -> Mux1/9  "Hall effect signal h_c"
  __UniqueInportName__10__/1 -> Mux1/10  "Rotor speed wm (rad/s)"
  __UniqueInportName__11__/1 -> Mux1/11  "Rotor angle thetam (rad)"
  __UniqueInportName__12__/1 -> Mux1/12  "Electromagnetic torque Te (N*m)"
  Mux1/1 -> motor_out/1

== system BLDCmotorControl_FOC_R2017b_fixdt/PWM_gates/PWM_generator1 ==
  DC : Inport  SampleTime=Ts
  PWM_generator_sfcn : S-Function  FunctionName=PWM_generator_sf  SFunctionModules=""  SFunctionDeploymentMode=off  EnableBusSupport=off  SFcnStateName=DWORK0  mask{rtw_sf_name=PWM_generator_sf, showVar=off}
      mask prompts: rtw_sf_name "Simulink:masks:GenSFuncName_MP"; showVar "Simulink:masks:GenSFuncShowModuleList_MP"
      mask help: Simulink:masks:GenSFuncDesc_MD
      mask init: same as BLDCmotorControl_FOC_R2017b_fixdt/BLDC_model_closed/BLDC_model_sfcn
      settings: SFcnIsStateOwnerBlock=on
      settings: CopyFcn=|
      | if ~strcmp(get_param(gcb,'Linkstatus'),'none') && ...
      | ~strcmp(get_param(gcb,'Linkstatus'),'implicit')
      |   set_param(gcb,'LinkStatus','none');
      | end
      mask Help: eval('feval(''rtwprivate'',''rtwhelpview'',''rtw_sfcn_block'')');
      mask Display:
      | port_label('input',1,'DC');
      | port_label('output',1,'PWM');
  __InputSSForSFun__ : Subsystem
  __OutputSSForSFun__ : Subsystem
  PWM : Outport
  wires:
  __OutputSSForSFun__/1(PWM) -> PWM/1
  PWM_generator_sfcn/1 -> __OutputSSForSFun__/1(__UniqueInportName__1__)
  __InputSSForSFun__/1(__UniqueOutportName__1__) -> PWM_generator_sfcn/1
  DC/1 -> __InputSSForSFun__/1(DC)

== system BLDCmotorControl_FOC_R2017b_fixdt/PWM_gates/PWM_generator12 ==
  DC : Inport  SampleTime=Ts
  PWM_generator_sfcn : S-Function  FunctionName=PWM_generator_sf  SFunctionModules=""  SFunctionDeploymentMode=off  EnableBusSupport=off  SFcnStateName=DWORK0  mask{rtw_sf_name=PWM_generator_sf, showVar=off}
      mask prompts: rtw_sf_name "Simulink:masks:GenSFuncName_MP"; showVar "Simulink:masks:GenSFuncShowModuleList_MP"
      mask help: Simulink:masks:GenSFuncDesc_MD
      mask init: same as BLDCmotorControl_FOC_R2017b_fixdt/BLDC_model_closed/BLDC_model_sfcn
      settings: SFcnIsStateOwnerBlock=on
      settings: CopyFcn=|
      | if ~strcmp(get_param(gcb,'Linkstatus'),'none') && ...
      | ~strcmp(get_param(gcb,'Linkstatus'),'implicit')
      |   set_param(gcb,'LinkStatus','none');
      | end
      mask Help: eval('feval(''rtwprivate'',''rtwhelpview'',''rtw_sfcn_block'')');
      mask Display:
      | port_label('input',1,'DC');
      | port_label('output',1,'PWM');
  __InputSSForSFun__ : Subsystem
  __OutputSSForSFun__ : Subsystem
  PWM : Outport
  wires:
  DC/1 -> __InputSSForSFun__/1(DC)
  __InputSSForSFun__/1(__UniqueOutportName__1__) -> PWM_generator_sfcn/1
  PWM_generator_sfcn/1 -> __OutputSSForSFun__/1(__UniqueInportName__1__)
  __OutputSSForSFun__/1(PWM) -> PWM/1

== system BLDCmotorControl_FOC_R2017b_fixdt/PWM_gates/PWM_generator2 ==
  DC : Inport  SampleTime=Ts
  PWM_generator_sfcn : S-Function  FunctionName=PWM_generator_sf  SFunctionModules=""  SFunctionDeploymentMode=off  EnableBusSupport=off  SFcnStateName=DWORK0  mask{rtw_sf_name=PWM_generator_sf, showVar=off}
      mask prompts: rtw_sf_name "Simulink:masks:GenSFuncName_MP"; showVar "Simulink:masks:GenSFuncShowModuleList_MP"
      mask help: Simulink:masks:GenSFuncDesc_MD
      mask init: same as BLDCmotorControl_FOC_R2017b_fixdt/BLDC_model_closed/BLDC_model_sfcn
      settings: SFcnIsStateOwnerBlock=on
      settings: CopyFcn=|
      | if ~strcmp(get_param(gcb,'Linkstatus'),'none') && ...
      | ~strcmp(get_param(gcb,'Linkstatus'),'implicit')
      |   set_param(gcb,'LinkStatus','none');
      | end
      mask Help: eval('feval(''rtwprivate'',''rtwhelpview'',''rtw_sfcn_block'')');
      mask Display:
      | port_label('input',1,'DC');
      | port_label('output',1,'PWM');
  __InputSSForSFun__ : Subsystem
  __OutputSSForSFun__ : Subsystem
  PWM : Outport
  wires:
  DC/1 -> __InputSSForSFun__/1(DC)
  __InputSSForSFun__/1(__UniqueOutportName__1__) -> PWM_generator_sfcn/1
  PWM_generator_sfcn/1 -> __OutputSSForSFun__/1(__UniqueInportName__1__)
  __OutputSSForSFun__/1(PWM) -> PWM/1

== system BLDCmotorControl_FOC_R2017b_fixdt/PWM_gates/PWM_generator3 ==
  DC : Inport  SampleTime=Ts
  PWM_generator_sfcn : S-Function  FunctionName=PWM_generator_sf  SFunctionModules=""  SFunctionDeploymentMode=off  EnableBusSupport=off  SFcnStateName=DWORK0  mask{rtw_sf_name=PWM_generator_sf, showVar=off}
      mask prompts: rtw_sf_name "Simulink:masks:GenSFuncName_MP"; showVar "Simulink:masks:GenSFuncShowModuleList_MP"
      mask help: Simulink:masks:GenSFuncDesc_MD
      mask init: same as BLDCmotorControl_FOC_R2017b_fixdt/BLDC_model_closed/BLDC_model_sfcn
      settings: SFcnIsStateOwnerBlock=on
      settings: CopyFcn=|
      | if ~strcmp(get_param(gcb,'Linkstatus'),'none') && ...
      | ~strcmp(get_param(gcb,'Linkstatus'),'implicit')
      |   set_param(gcb,'LinkStatus','none');
      | end
      mask Help: eval('feval(''rtwprivate'',''rtwhelpview'',''rtw_sfcn_block'')');
      mask Display:
      | port_label('input',1,'DC');
      | port_label('output',1,'PWM');
  __InputSSForSFun__ : Subsystem
  __OutputSSForSFun__ : Subsystem
  PWM : Outport
  wires:
  __OutputSSForSFun__/1(PWM) -> PWM/1
  PWM_generator_sfcn/1 -> __OutputSSForSFun__/1(__UniqueInportName__1__)
  __InputSSForSFun__/1(__UniqueOutportName__1__) -> PWM_generator_sfcn/1
  DC/1 -> __InputSSForSFun__/1(DC)

== system BLDCmotorControl_FOC_R2017b_fixdt/PWM_gates/PWM_generator4 ==
  DC : Inport  SampleTime=Ts
  PWM_generator_sfcn : S-Function  FunctionName=PWM_generator_sf  SFunctionModules=""  SFunctionDeploymentMode=off  EnableBusSupport=off  SFcnStateName=DWORK0  mask{rtw_sf_name=PWM_generator_sf, showVar=off}
      mask prompts: rtw_sf_name "Simulink:masks:GenSFuncName_MP"; showVar "Simulink:masks:GenSFuncShowModuleList_MP"
      mask help: Simulink:masks:GenSFuncDesc_MD
      mask init: same as BLDCmotorControl_FOC_R2017b_fixdt/BLDC_model_closed/BLDC_model_sfcn
      settings: SFcnIsStateOwnerBlock=on
      settings: CopyFcn=|
      | if ~strcmp(get_param(gcb,'Linkstatus'),'none') && ...
      | ~strcmp(get_param(gcb,'Linkstatus'),'implicit')
      |   set_param(gcb,'LinkStatus','none');
      | end
      mask Help: eval('feval(''rtwprivate'',''rtwhelpview'',''rtw_sfcn_block'')');
      mask Display:
      | port_label('input',1,'DC');
      | port_label('output',1,'PWM');
  __InputSSForSFun__ : Subsystem
  __OutputSSForSFun__ : Subsystem
  PWM : Outport
  wires:
  DC/1 -> __InputSSForSFun__/1(DC)
  __InputSSForSFun__/1(__UniqueOutportName__1__) -> PWM_generator_sfcn/1
  PWM_generator_sfcn/1 -> __OutputSSForSFun__/1(__UniqueInportName__1__)
  __OutputSSForSFun__/1(PWM) -> PWM/1

== system BLDCmotorControl_FOC_R2017b_fixdt/PWM_gates/PWM_generator5 ==
  DC : Inport  SampleTime=Ts
  PWM_generator_sfcn : S-Function  FunctionName=PWM_generator_sf  SFunctionModules=""  SFunctionDeploymentMode=off  EnableBusSupport=off  SFcnStateName=DWORK0  mask{rtw_sf_name=PWM_generator_sf, showVar=off}
      mask prompts: rtw_sf_name "Simulink:masks:GenSFuncName_MP"; showVar "Simulink:masks:GenSFuncShowModuleList_MP"
      mask help: Simulink:masks:GenSFuncDesc_MD
      mask init: same as BLDCmotorControl_FOC_R2017b_fixdt/BLDC_model_closed/BLDC_model_sfcn
      settings: SFcnIsStateOwnerBlock=on
      settings: CopyFcn=|
      | if ~strcmp(get_param(gcb,'Linkstatus'),'none') && ...
      | ~strcmp(get_param(gcb,'Linkstatus'),'implicit')
      |   set_param(gcb,'LinkStatus','none');
      | end
      mask Help: eval('feval(''rtwprivate'',''rtwhelpview'',''rtw_sfcn_block'')');
      mask Display:
      | port_label('input',1,'DC');
      | port_label('output',1,'PWM');
  __InputSSForSFun__ : Subsystem
  __OutputSSForSFun__ : Subsystem
  PWM : Outport
  wires:
  __OutputSSForSFun__/1(PWM) -> PWM/1
  PWM_generator_sfcn/1 -> __OutputSSForSFun__/1(__UniqueInportName__1__)
  __InputSSForSFun__/1(__UniqueOutportName__1__) -> PWM_generator_sfcn/1
  DC/1 -> __InputSSForSFun__/1(DC)

== system BLDCmotorControl_FOC_R2017b_fixdt/PWM_gates/signal_log6 ==
  PWM : Inport
  Terminator_1 : Terminator
  wires:
  PWM/1 -> Terminator_1/1  "PWM"

== system BLDCmotorControl_FOC_R2017b_fixdt/filtLowPass/Low_Pass_Filter ==
  u : Inport
  coef : Inport  Port=2
  Divide3 : Product  Inputs=**  OutDataTypeStr=fixdt(1,32,16)  RndMeth=Simplest  SaturateOnIntegerOverflow=on
  Scope1 : Scope  NumInputPorts=3
  Sum2 : Sum  Inputs=+-  RndMeth=Simplest
  Sum3 : Sum  RndMeth=Simplest  OutDataTypeStr=Inherit: Same as first input
  UnitDelay1 : UnitDelay  SampleTime=-1
  y : Outport
  wires:
  Divide3/1 -> Scope1/2, Sum3/1
  Sum3/1 -> y/1, Scope1/3, UnitDelay1/1
  UnitDelay1/1 -> Sum3/2, Sum2/2
  Sum2/1 -> Divide3/1, Scope1/1
  u/1 -> Sum2/1
  coef/1 -> Divide3/2

== system BLDCmotorControl_FOC_R2017b_fixdt/rateLimiter/Rate_Limiter ==
  note: Rate Limiter
      | Note: The sample time must be included in the Increment and Decrement values.
  u : Inport
  inc : Inport  Port=2
  dec : Inport  Port=3
  Saturation Dynamic : simulink/Discontinuities/Saturation Dynamic  OutMin=[]  OutMax=[]  OutDataTypeStr=Inherit: Same as second input  OutDataType=fixdt(1, 16)  OutScaling=2^-10  DoSatur=off
  Sum1 : Sum  Inputs=+-  RndMeth=Zero  OutDataTypeStr=Inherit: Same as first input
  Sum2 : Sum  RndMeth=Zero  OutDataTypeStr=Inherit: Same as first input
  UnitDelay : UnitDelay  SampleTime=-1
      settings: AttributesFormatString=Ini=%<X0>
  y : Outport
  wires:
  Saturation Dynamic/1 -> Sum2/1
  dec/1 -> Saturation Dynamic/3
  Sum1/1 -> Saturation Dynamic/2
  Sum2/1 -> UnitDelay/1, y/1
  inc/1 -> Saturation Dynamic/1
  u/1 -> Sum1/1
  UnitDelay/1 -> Sum2/2, Sum1/2

== system BLDCmotorControl_FOC_R2017b_fixdt/BLDC_controller/F01_Estimations/F01_01_Edge_Detector ==
  b_hallA : Inport
  b_hallB : Inport  Port=2
  b_hallC : Inport  Port=3
  Logical Operator : Logic  Operator=XOR  Inputs=6  AllPortsSameDT=off  OutDataTypeStr=boolean
  UnitDelay1 : UnitDelay  SampleTime=-1
      settings: AttributesFormatString=Ini=%<X0>
  UnitDelay2 : UnitDelay  SampleTime=-1
      settings: AttributesFormatString=Ini=%<X0>
  UnitDelay3 : UnitDelay  SampleTime=-1
      settings: AttributesFormatString=Ini=%<X0>
  "b_edge " : Outport  OutputWhenDisabled=reset  InitialOutput=0
  wires:
  b_hallA/1 -> Logical Operator/1, UnitDelay3/1
  b_hallC/1 -> Logical Operator/3, UnitDelay2/1
  b_hallB/1 -> Logical Operator/2, UnitDelay1/1
  UnitDelay1/1 -> Logical Operator/5
  UnitDelay2/1 -> Logical Operator/6
  UnitDelay3/1 -> Logical Operator/4
  Logical Operator/1 -> "b_edge "/1

== system BLDCmotorControl_FOC_R2017b_fixdt/BLDC_controller/F01_Estimations/F01_02_Position_Calculation ==
  note: This calculates the low resolution position based on Hall sensors.
  b_hallA : Inport
  b_hallB : Inport  Port=2
  b_hallC : Inport  Port=3
  Selector : Selector  IndexMode=Zero-based  InputPortWidth=length(vec_hallToPos)  IndexOptions=Index vector (port)  Indices=[1 3]  OutputSizes=1
  Sum : Sum  Inputs=+++  RndMeth=Simplest  OutDataTypeStr=Inherit: Same as first input
  g_Ha : Gain  Gain=4  OutDataTypeStr=Inherit: Inherit via back propagation  RndMeth=Zero  ParamDataTypeStr=Inherit: Same as input
  g_Hb : Gain  Gain=2  OutDataTypeStr=Inherit: Inherit via back propagation  RndMeth=Simplest  ParamDataTypeStr=Inherit: Same as input
  vec_hallToPos : Constant  Value=vec_hallToPos  OutDataTypeStr=int8
  z_posRaw : Outport  OutputWhenDisabled=reset  InitialOutput=0
  "z_pos " : Outport  Port=2  OutputWhenDisabled=reset  InitialOutput=0
  wires:
  b_hallC/1 -> Sum/3
  g_Ha/1 -> Sum/1
  g_Hb/1 -> Sum/2
  Sum/1 -> z_posRaw/1, Selector/2
  b_hallA/1 -> g_Ha/1
  b_hallB/1 -> g_Hb/1
  vec_hallToPos/1 -> Selector/1
  Selector/1 -> "z_pos "/1

== system BLDCmotorControl_FOC_R2017b_fixdt/BLDC_controller/F01_Estimations/F01_03_Direction_Detection ==
  z_pos : Inport
  Action Port : ActionPort  ActionType=then
  Constant20 : Constant  Value=-5  OutDataTypeStr=Inherit: Inherit via back propagation
  Constant23 : Constant  Value=-1  OutDataTypeStr=int8
  Constant24 : Constant  OutDataTypeStr=int8
  Constant8 : Constant  OutDataTypeStr=Inherit: Inherit via back propagation
  Logical Operator3 : Logic  Operator=OR  AllPortsSameDT=off  OutDataTypeStr=boolean
  Relational Operator1 : RelationalOperator  Operator===  OutDataTypeStr=boolean  RndMeth=Simplest
  Relational Operator6 : RelationalOperator  Operator===  OutDataTypeStr=boolean  RndMeth=Simplest
  Sum2 : Sum  Inputs=|+-  RndMeth=Zero  InputSameDT=on  OutDataTypeStr=Inherit: Same as first input
  Switch2 : Switch  Criteria=u2 ~= 0  OutDataTypeStr=Inherit: Inherit via back propagation  RndMeth=Simplest
  UnitDelay2 : UnitDelay  SampleTime=-1
  UnitDelay3 : UnitDelay  SampleTime=-1
      settings: AttributesFormatString=Ini=%<X0>
  z_dir : Outport
  z_dirPrev : Outport  Port=2
  wires:
  UnitDelay2/1 -> Sum2/2
  Relational Operator1/1 -> Logical Operator3/1
  Constant8/1 -> Relational Operator1/2
  Sum2/1 -> Relational Operator6/1, Relational Operator1/1
  Relational Operator6/1 -> Logical Operator3/2
  Constant20/1 -> Relational Operator6/2
  Constant24/1 -> Switch2/1
  Constant23/1 -> Switch2/3
  Logical Operator3/1 -> Switch2/2
  z_pos/1 -> Sum2/1, UnitDelay2/1
  Switch2/1 -> UnitDelay3/1, z_dir/1
  UnitDelay3/1 -> z_dirPrev/1

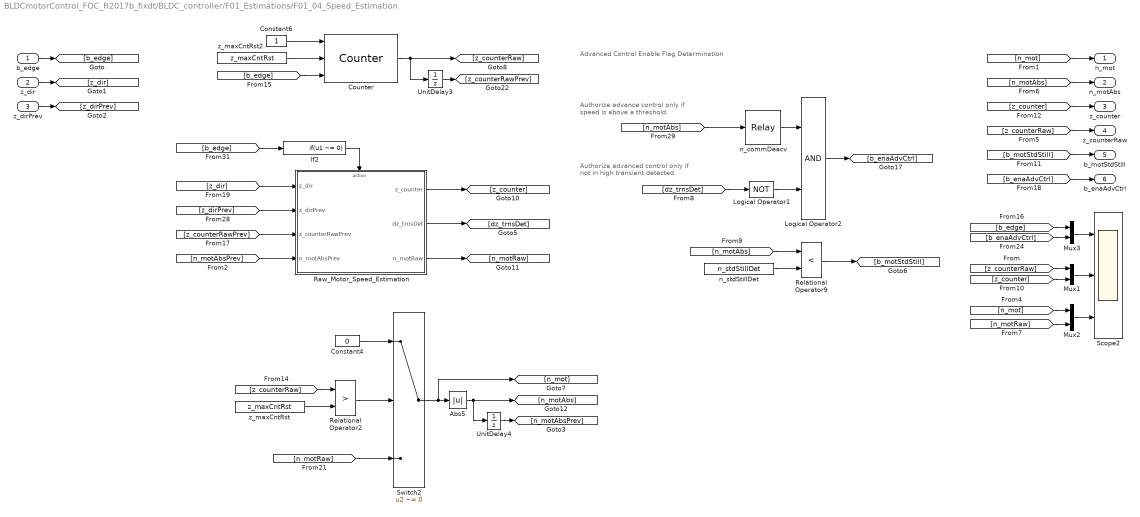
== system BLDCmotorControl_FOC_R2017b_fixdt/BLDC_controller/F01_Estimations/F01_04_Speed_Estimation ==
  note: Advanced Control Enable Flag Determination
  note: Authorize advance control only if speed is above a threshold.
  note: Authorize advanced control only if not in high transient detected.
  b_edge : Inport
  z_dir : Inport  Port=2
  z_dirPrev : Inport  Port=3
  Abs5 : Abs  OutDataTypeStr=Inherit: Inherit via back propagation  RndMeth=Zero
  Constant4 : Constant  Value=0  OutDataTypeStr=Inherit: Inherit via back propagation
  Constant6 : Constant  OutDataTypeStr=fixdt(1,16,0)
  Counter : BLDC_controller_Lib/Counter  z_cntInit=z_maxCntRst
      settings: AttributesFormatString=Ini=%<z_cntInit>
  If2 : If  IfExpression=u1 ~= 0  ShowElse=off
  Logical Operator1 : Logic  Operator=NOT  AllPortsSameDT=off  OutDataTypeStr=boolean
  Logical Operator2 : Logic  AllPortsSameDT=off  OutDataTypeStr=boolean
  Mux1 : Mux  Inputs=2
  Mux2 : Mux  Inputs=2
  Mux3 : Mux  Inputs=2
  Raw_Motor_Speed_Estimation : Subsystem
  Relational Operator2 : RelationalOperator  Operator=>  OutDataTypeStr=boolean  RndMeth=Simplest
  Relational Operator9 : RelationalOperator  Operator=<  OutDataTypeStr=boolean  RndMeth=Simplest
  Scope2 : Scope  NumInputPorts=3
  Switch2 : Switch  Criteria=u2 ~= 0  OutDataTypeStr=Inherit: Inherit via back propagation  RndMeth=Zero
  UnitDelay3 : UnitDelay  InitialCondition=z_maxCntRst  SampleTime=-1
      settings: AttributesFormatString=Ini=%<X0>
  UnitDelay4 : UnitDelay  SampleTime=-1
      settings: AttributesFormatString=Ini=%<X0>
  n_commDeacv : Relay  OnSwitchValue=n_commDeacvHi  OffSwitchValue=n_commAcvLo  OutDataTypeStr=boolean
  n_stdStillDet : Constant  Value=n_stdStillDet  OutDataTypeStr=Inherit: Inherit via back propagation
  z_maxCntRst : Constant  Value=z_maxCntRst  OutDataTypeStr=Inherit: Inherit via back propagation
  z_maxCntRst2 : Constant  Value=z_maxCntRst  OutDataTypeStr=Inherit: Inherit via back propagation
  n_mot : Outport
  n_motAbs : Outport  Port=2
  z_counter : Outport  Port=3  OutputWhenDisabled=reset  InitialOutput=0
  z_counterRaw : Outport  Port=4  OutputWhenDisabled=reset  InitialOutput=0
  b_motStdStill : Outport  Port=5  OutputWhenDisabled=reset  InitialOutput=0
  b_enaAdvCtrl : Outport  Port=6
  wires:
  [n_motRaw] -> Mux2/2
  Mux2/1 -> Scope2/3
  [n_mot] -> Mux2/1
  Mux1/1 -> Scope2/2
  [z_counterRaw] -> Mux1/1
  [z_counter] -> Mux1/2
  b_edge/1 -> [b_edge]
  [n_mot] -> n_mot/1
  z_dir/1 -> [z_dir]
  [z_counter] -> z_counter/1
  [z_counterRaw] -> z_counterRaw/1
  UnitDelay3/1 -> [z_counterRawPrev]
  z_dirPrev/1 -> [z_dirPrev]
  [z_dir] -> Raw_Motor_Speed_Estimation/1(z_dir)
  Abs5/1 -> UnitDelay4/1, [n_motAbs]
  Raw_Motor_Speed_Estimation/1(z_counter) -> [z_counter]
  [z_dirPrev] -> Raw_Motor_Speed_Estimation/2(z_dirPrev)
  If2/1 -> Raw_Motor_Speed_Estimation/Action
  [z_counterRawPrev] -> Raw_Motor_Speed_Estimation/3(z_counterRawPrev)
  [b_enaAdvCtrl] -> b_enaAdvCtrl/1
  [z_counterRaw] -> Relational Operator2/1
  z_maxCntRst/1 -> Relational Operator2/2
  Constant4/1 -> Switch2/1
  Raw_Motor_Speed_Estimation/3(n_motRaw) -> [n_motRaw]
  Switch2/1 -> [n_mot], Abs5/1
  Mux3/1 -> Scope2/1
  [b_enaAdvCtrl] -> Mux3/2
  [b_edge] -> Mux3/1
  [b_edge] -> If2/1
  Relational Operator2/1 -> Switch2/2
  UnitDelay4/1 -> [n_motAbsPrev]
  [n_motAbsPrev] -> Raw_Motor_Speed_Estimation/4(n_motAbsPrev)
  [n_motAbs] -> n_motAbs/1
  [n_motAbs] -> n_commDeacv/1
  Raw_Motor_Speed_Estimation/2(dz_trnsDet) -> [dz_trnsDet]
  n_commDeacv/1 -> Logical Operator2/1
  Logical Operator1/1 -> Logical Operator2/2
  Logical Operator2/1 -> [b_enaAdvCtrl]
  [dz_trnsDet] -> Logical Operator1/1
  z_maxCntRst2/1 -> Counter/2
  [b_edge] -> Counter/3
  Constant6/1 -> Counter/1
  Counter/1 -> UnitDelay3/1, [z_counterRaw]
  [b_motStdStill] -> b_motStdStill/1
  [n_motAbs] -> Relational Operator9/1
  n_stdStillDet/1 -> Relational Operator9/2
  Relational Operator9/1 -> [b_motStdStill]
  [n_motRaw] -> Switch2/3
